simulink model "QAMV2"  (R2024b)
settings: Solver=VariableStepAuto  StartTime=0.0  StopTime=5  RelTol=1e-3
libraries: simulink x4, simulink_extras x3, commdigbbndam3 x2, dspvision x1
settings Model: LastModifiedBy=fredy

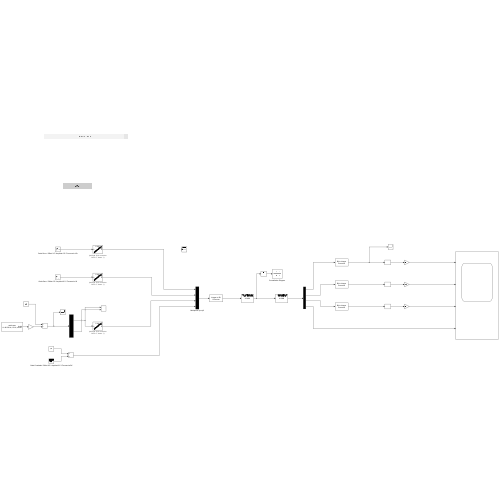
[thumbnail: Simulink's stored preview of the top-level diagram]
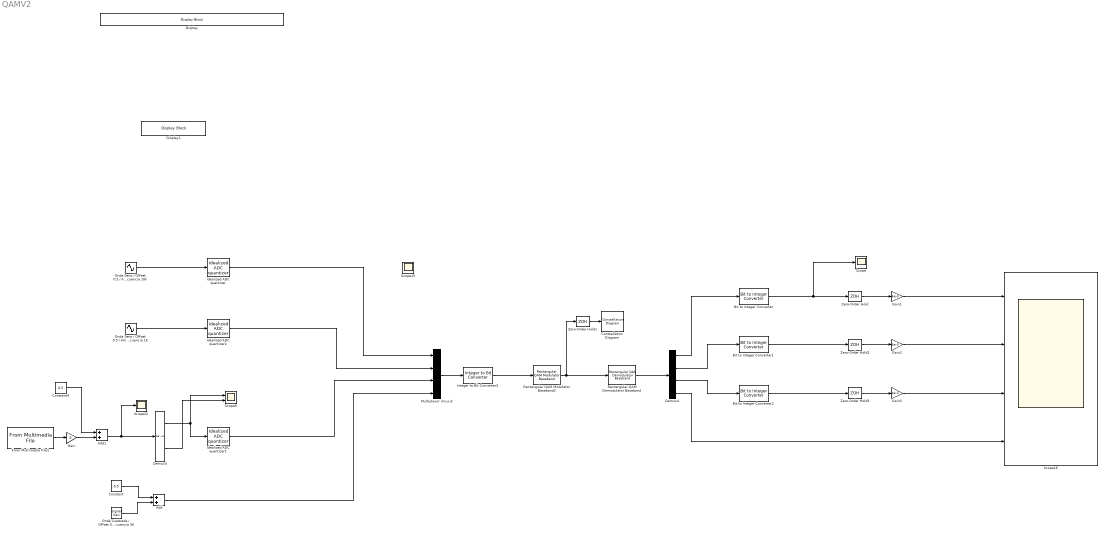
== system QAMV2 ==
  Add : Sum
  Add1 : Sum
  Bit to Integer Converter : simulink/Logic and Bit Operations/Bit to Integer Converter  nbits=8  bitOrder=MSB first  signedOutputValues=Unsigned  outDtype=Inherit via internal rule  outDtypeSigned=Inherit via internal rule
  Bit to Integer Converter1 : simulink/Logic and Bit Operations/Bit to Integer Converter  nbits=8  bitOrder=MSB first  signedOutputValues=Unsigned  outDtype=Inherit via internal rule  outDtypeSigned=Inherit via internal rule
  Bit to Integer Converter2 : simulink/Logic and Bit Operations/Bit to Integer Converter  nbits=8  bitOrder=MSB first  signedOutputValues=Unsigned  outDtype=Inherit via internal rule  outDtypeSigned=Inherit via internal rule
  Constant : Constant  Value=0.5
  Constant4 : Constant  Value=0.5
  Constellation Diagram : ConstellationDiagram  WindowPosition=[373.000000,675.000000,600.000000,600.000000,]  Visible=on  ScopeFrameLocation=window
  Demux4 : Demux
  Demux5 : Demux  Outputs=2
  Display : DisplayBlock  LabelPosition=Hide  Transparency=1  Layout=Fill available space
  Display1 : DisplayBlock  LabelPosition=Hide  Transparency=1
  From Multimedia File1 : dspvision/From Multimedia File  inputFilename=D:\Datos Fredy\Programacion\Matlab\Modulacion ASK\audio.wav  readRange=[1 Inf]  loop=on  numPlays=inf  outputStreams=Audio only  videoDataType=single  audioDataType=single  inheritSampleTime=on  userDefinedSampleTime=1/30  noAudioOutput=off  isIntensityVideo=off  fourcc=RGB  colorVideoFormat=Separate color signals  outputEOF=off  dataOrg=Column-major  audioFrameSize=1  computeAudioFrameSize=off  outSamplingMode=Sample based
      settings: LibrarySourceBlock=audiosources/From Multimedia File
  Gain : Gain  Gain=.5
  Gain1 : Gain  Gain=4e-3
  Gain2 : Gain  Gain=4e-3
  Gain3 : Gain  Gain=4e-3
  Idealized ADC quantizer : simulink_extras/Additional Discrete/Idealized ADC quantizer  NumberOfConverterBits=8  Vmin=0  Vmax=1  OutputDataType=double  OutputNegativeValues=off
  Idealized ADC quantizer1 : simulink_extras/Additional Discrete/Idealized ADC quantizer  NumberOfConverterBits=8  Vmin=0  Vmax=1  OutputDataType=double  OutputNegativeValues=off
  Idealized ADC quantizer2 : simulink_extras/Additional Discrete/Idealized ADC quantizer  NumberOfConverterBits=8  Vmin=0  Vmax=1  OutputDataType=double  OutputNegativeValues=off
  Integer to Bit Converter3 : simulink/Logic and Bit Operations/Integer to Bit Converter  nbits=8  signedInputValues=Unsigned  bitOrder=MSB first  outDtype=Inherit via internal rule
  Multiplexor (mux)2 : Mux
  Onda Cuadrada / Offset 0.5 / Amplitud 0.5 / Frecuencia 5K : SignalGenerator  WaveForm=square  Amplitude=0.5  Frequency=5000
  Onda Seno / Offset 0.5 / Amplitud 0.5 / Frecuencia 10k : Sin  Amplitude=0.5  Bias=0.5  Frequency=62831.853071  SampleTime=0
  Onda Seno / Offset 0.5 / Amplitud 0.5 / Frecuencia 1K : Sin  Amplitude=0.5  Bias=0.5  Frequency=6283.185307  SampleTime=0
  Rectangular QAM Demodulator Baseband : commdigbbndam3/Rectangular QAM Demodulator Baseband  M=4  OutType=Bit  DecType=Hard decision  VarSource=Dialog  Variance=1  Dec=Gray  Mapping=[0:15]  PowType=Average Power  MinDist=4  AvgPow=1  PeakPow=1  Ph=0  outDtype1=Inherit via internal rule  outDtype2=Inherit via internal rule  derotateFactorWordLen=16  derotateFactorDataTypeStr=Inherit: Same word length as input  derotateFactorLastDataTypeStr=Inherit: Same word length as input  denormFactorWordLen=16  denormFactorDataTypeStr=Inherit: Same word length as input  denormFactorLastDataTypeStr=Inherit: Same word length as input  prodOutWordLen=32  prodOutOverflowMode=Wrap  prodOutRoundingMode=Floor  prodOutOvFlMode=off  prodOutOvFlModeLastStrValue=off  sumWordLen=32
      settings: LibrarySourceBlock=|
      | commhdldigbbndam/Rectangular QAM
      | Demodulator
      | Baseband
  Rectangular QAM Modulator Baseband2 : commdigbbndam3/Rectangular QAM Modulator Baseband  M=4  InType=Bit  Enc=Gray  Mapping=[0:15]  PowType=Average Power  MinDist=4  AvgPow=1  PeakPow=1  Ph=0  outDtype=double  outWordLen=16  outUDDataType=sfix(16)  outFracLenMode=Best precision  outFracLen=15  outDataTypeStr=double  outLastDataTypeStr=double
      settings: LibrarySourceBlock=|
      | commhdldigbbndam/Rectangular QAM
      | Modulator
      | Baseband
  Scope : Scope
  Scope15 : Scope
  Scope16 : Scope  NumInputPorts=4
  Scope22 : Scope
  Scope9 : Scope  NumInputPorts=2
  Zero-Order Hold : ZeroOrderHold  SampleTime=-1
  Zero-Order Hold1 : ZeroOrderHold  SampleTime=0.0001
  Zero-Order Hold2 : ZeroOrderHold  SampleTime=-1
  Zero-Order Hold3 : ZeroOrderHold  SampleTime=-1
  wires:
  Constant/1 -> Add/1
  Onda Cuadrada / Offset 0.5 / Amplitud 0.5 / Frecuencia 5K/1 -> Add/2
  Idealized ADC quantizer2/1 -> Multiplexor (mux)2/2
  Constant4/1 -> Add1/1
  Onda Seno / Offset 0.5 / Amplitud 0.5 / Frecuencia 1K/1 -> Idealized ADC quantizer2/1
  Bit to Integer Converter1/1 -> Zero-Order Hold2/1
  Bit to Integer Converter2/1 -> Zero-Order Hold3/1
  Add1/1 -> Scope22/1, Demux5/1
  From Multimedia File1/1 -> Gain/1
  Gain/1 -> Add1/2
  Demux5/1 -> Scope9/1, Idealized ADC quantizer1/1
  Demux5/2 -> Scope9/2
  Idealized ADC quantizer1/1 -> Multiplexor (mux)2/3
  Add/1 -> Multiplexor (mux)2/4
  Onda Seno / Offset 0.5 / Amplitud 0.5 / Frecuencia 10k/1 -> Idealized ADC quantizer/1
  Idealized ADC quantizer/1 -> Multiplexor (mux)2/1
  Multiplexor (mux)2/1 -> Integer to Bit Converter3/1
  Integer to Bit Converter3/1 -> Rectangular QAM Modulator Baseband2/1
  Rectangular QAM Modulator Baseband2/1 -> Zero-Order Hold1/1, Rectangular QAM Demodulator Baseband/1
  Rectangular QAM Demodulator Baseband/1 -> Demux4/1
  Demux4/3 -> Bit to Integer Converter2/1
  Demux4/2 -> Bit to Integer Converter1/1
  Demux4/1 -> Bit to Integer Converter/1
  Demux4/4 -> Scope16/4
  Zero-Order Hold1/1 -> Constellation Diagram/1
  Zero-Order Hold/1 -> Gain1/1
  Bit to Integer Converter/1 -> Scope/1, Zero-Order Hold/1
  Zero-Order Hold2/1 -> Gain2/1
  Zero-Order Hold3/1 -> Gain3/1
  Gain1/1 -> Scope16/1
  Gain2/1 -> Scope16/2
  Gain3/1 -> Scope16/3
